simulink model "elevation_gyro_PLANT"  (R2022a)
settings: Solver=VariableStepAuto  StartTime=0.0  StopTime=5  RelTol=1e-3
model workspace (MAT data in the model file):
  elevation_gyro_plant.g = [-51.237663269 -52.0182609558 -52.1288909912 -52.6638412476 -53.0468559265 -53.6800422668 -53.6302185059 -54.005317688 -54.5245552063 -54.9788475037 -55.300819397 -55.6738739014 ... (985 elements, 1x985)]
  elevation_gyro_plant.o2i1 = [0.00107155356091-0.00252429093234i 0.000947028165683-0.00232082675211i 0.000882330641616-0.00231226254255i 0.000830446369946-0.00217383913696i 0.000775892985985-0.00208712229505i 0.000701846380252-0.00194752507377i 0.00068766286131-0.00196519983001i 0.000640989514068-0.00188820890617i 0.000582222943194-0.00178581802174i 0.000550608965568-0.00169544888195i 0.000524186645634-0.00163581233937i 0.000497277767863-0.0015685944818i ... (985 elements, 1x985)]
  elevation_gyro_plant.o2i1x = [3 3.20000004768 3.40000009537 3.59999990463 3.79999995232 4 4.19999980927 4.40000009537 4.59999990463 4.80000019073 5 5.19999980927 ... (985 elements, 1x985)]
  elevation_gyro_plant.p = [-66.9989318848 -67.8017730713 -69.1137695312 -69.0922241211 -69.6072540283 -70.1819229126 -70.7140350342 -71.2492141724 -71.9426879883 -72.008430481 -72.2322387695 -72.4102783203 ... (985 elements, 1x985)]
undefined symbols (not defined in the file or in its folder): fix_conseg, JLreg, JMreg, Kkeg, Kveg
libraries: slctrlblks x1
settings Model: Creator=ohadformanair  LastModifiedBy=ohadformanair
settings SolverCC: ZeroCrossAlgorithm=Adaptive
settings DebuggingCC: IgnoredZcDiagnostic=none

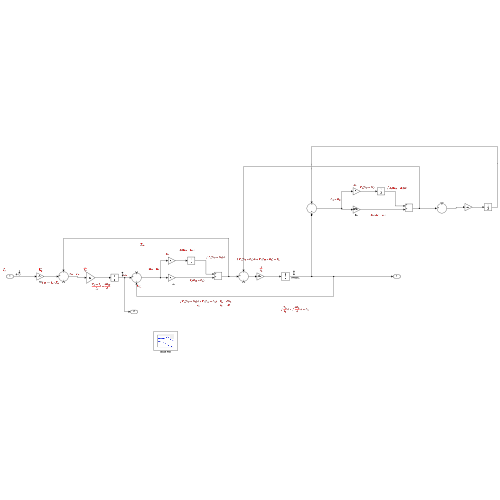
[thumbnail: Simulink's stored preview of the top-level diagram]
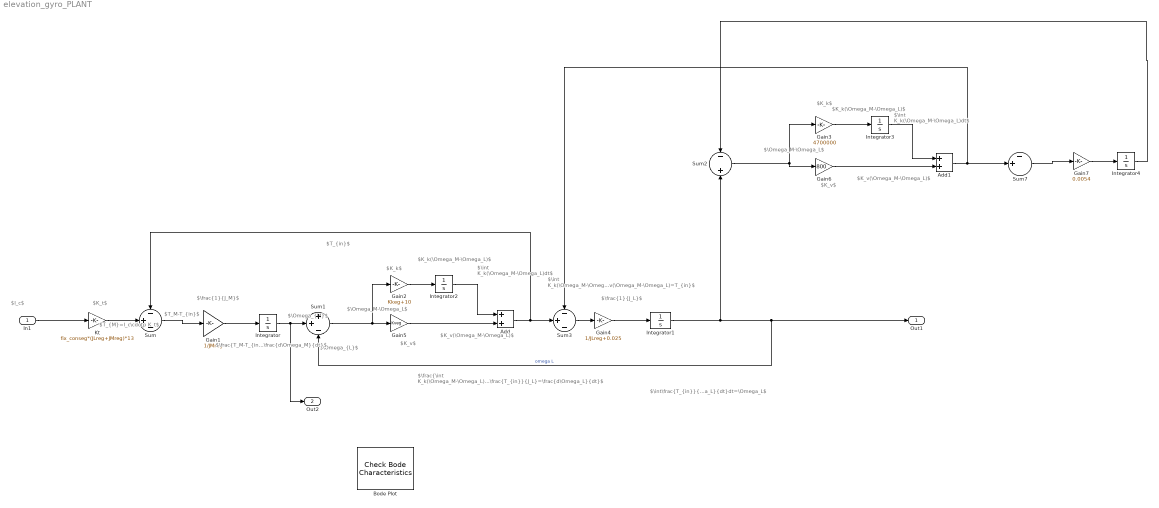
== system elevation_gyro_PLANT ==
  note: $\int\frac{T_{in}}{J_L}dt=\int\frac{d\Omega_L}{dt}dt=\Omega_L$
  note: $\Omega_M-\Omega_L$
  note: $\Omega_{L}$
  note: $K_k(\Omega_M-\Omega_L)$
  note: $\frac{1}{J_L}$
  note: $\int K_k(\Omega_M-\Omega_L)dt+K_v(\Omega_M-\Omega_L)=T_{in}$
  note: $T_{M}=I_c\cdotp K_t$
  note: $T_M-T_{in}$
  note: $K_v(\Omega_M-\Omega_L)$
  note: $\int K_k(\Omega_M-\Omega_L)dt$
  note: $K_v$
  note: $K_k$
  note: $T_{in}$
  note: $K_k(\Omega_M-\Omega_L)$
  note: $K_v$
  note: $K_k$
  note: $\int K_k(\Omega_M-\Omega_L)dt$
  note: $\frac{1}{J_M}$
  note: $\Omega_M-\Omega_L$
  note: $\Omega_{M}$
  note: $K_t$
  note: $I_c$
  note: $\frac{\int K_k(\Omega_M-\Omega_L)dt+K_v(\Omega_M-\Omega_L)}{J_L}=\frac{T_{in}}{J_L}=\frac{d\Omega_L}{dt}$
  note: $\frac{T_M-T_{in}}{J_M}=\frac{d\Omega_M}{dt}$
  note: $K_v(\Omega_M-\Omega_L)$
  In1 : Inport
  Add : Sum
  Add1 : Sum
  Bode Plot : slctrlblks/Model Verification/Check Bode  Characteristics  InstantiateOnLoad=on  SaveOperatingPoints=off  LinearizationIOs={'/In1', 1, 'in', 'off', '';'/Integrator', 1, 'out', 'off', ''}  LinearizeAt=SnapshotTimes  SnapshotTimes=[0]  TriggerType=rising  SampleTime=auto  RateConversionMethod=zoh  PreWarpFreq=10  UseExactDelayModel=off  UseFullBlockNameLabels=off  UseBusSignalLabels=off  enabled=on  stopWhenAssertionFail=off  export=off  ViewDlgPos=[25 318 650 502]  OpenViewOnLoad=off  LaunchViewOnOpen=off  FrequencyUnits=Hz  MagnitudeUnits=dB  PhaseUnits=deg  TimeUnits=seconds  EnableUpperBound=off  UpperBoundFrequencies=[]  UpperBoundMagnitudes=[]  EnableLowerBound=off  LowerBoundFrequencies=[]  LowerBoundMagnitudes=[]
  Gain1 : Gain  Gain=1/JMreg
  Gain2 : Gain  Gain=Kkeg+10
  Gain3 : Gain  Gain=4700000
  Gain4 : Gain  Gain=1/JLreg+0.025
  Gain5 : Gain  Gain=Kveg
  Gain6 : Gain  Gain=800
  Gain7 : Gain  Gain=0.0054
  Integrator{,1..4} (5 alike) : Integrator
  Kt : Gain  Gain=fix_conseg*(JLreg+JMreg)*13
  Sum : Sum  Inputs=-+-
  Sum1 : Sum  Inputs=++-
  Sum2 : Sum  Inputs=-+
  Sum3 : Sum  Inputs=-+-
  Sum7 : Sum  Inputs=-+|
  Out1 : Outport
  Out2 : Outport  Port=2
  wires:
  Gain1/1 -> Integrator/1
  Add/1 -> Sum3/2, Sum/1
  Gain3/1 -> Integrator3/1
  Kt/1 -> Sum/2
  Gain7/1 -> Integrator4/1
  Sum2/1 -> Gain6/1, Gain3/1
  Sum/1 -> Gain1/1
  Gain6/1 -> Add1/2
  Gain4/1 -> Integrator1/1
  Add1/1 -> Sum3/1, Sum7/2
  Sum3/1 -> Gain4/1
  Integrator2/1 -> Add/1
  Gain2/1 -> Integrator2/1
  Integrator3/1 -> Add1/1
  Integrator/1 -> Out2/1, Sum1/2
  Gain5/1 -> Add/2
  Sum1/1 -> Gain5/1, Gain2/1
  Integrator1/1 -> Sum1/3, Out1/1, Sum2/2  "omega L"
  Integrator4/1 -> Sum2/1
  Sum7/1 -> Gain7/1
  In1/1 -> Kt/1
